simulink model "example_transient_pemfc"  (R2025a)
settings: Solver=ode15s  StartTime=0.0  StopTime=300  RelTol=1e-3
InitFcn:
  | pyenv_setup(); create_buses(5);
model workspace (MAT data in the model file):
  anFlowStruct.temperature = 344.15
  anFlowStruct.pressure = 190000
  anFlowStruct.o2 = 0
  anFlowStruct.n2 = 0
  anFlowStruct.h2 = 3.62749438e-07
  anFlowStruct.h2o = 3.83749167e-08
  anFlowStruct.liquid = 0
  caFlowStruct.temperature = 344.15
  caFlowStruct.pressure = 140000
  caFlowStruct.o2 = 2.07285393e-07
  caFlowStruct.n2 = 7.79787907e-07
  caFlowStruct.h2 = 0
  caFlowStruct.h2o = 6.4862692e-08
  caFlowStruct.liquid = 0
values from neighbouring files (symbols this model uses):
  anFlowStruct = struct('temperature', 344.15, 'pressure', 190000.,          'o2', 0., 'n2', 0., 'h2', 3.62749438e-7, 'h2o', 3.83749167e-8, 'liquid', 0.)    [build_example_transient_pemfc.m]    (also in build_transient_block.m = struct('temperature', 344.15, 'pressure', 190000.,          )
  caFlowStruct = struct('temperature', 344.15, 'pressure', 140000.,          'o2', 2.07285393e-7, 'n2', 7.79787907e-7, 'h2', 0., 'h2o', 6.48626920e-8, 'liquid', 0.)    [build_example_transient_pemfc.m]    (also in build_transient_block.m = struct('temperature', 344.15, 'pressure', 140000.,          )
settings Model: Creator=paffonsonobrega  LastModifiedBy=paffonsonobrega

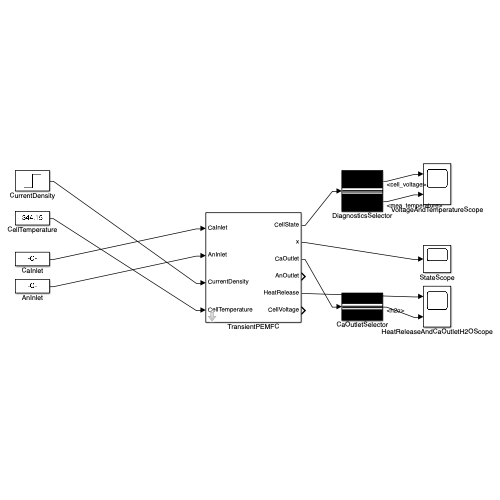
[thumbnail: Simulink's stored preview of the top-level diagram]
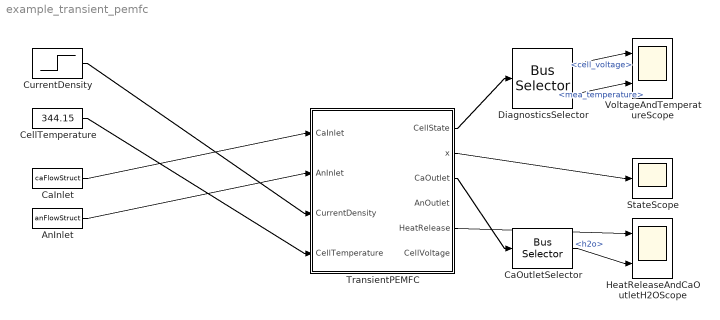
== system example_transient_pemfc ==
  AnInlet : Constant  Value=anFlowStruct  OutDataTypeStr=Bus: GasFlowStateBus
  CaInlet : Constant  Value=caFlowStruct  OutDataTypeStr=Bus: GasFlowStateBus
  CaOutletSelector : BusSelector  OutputSignals=h2o
  CellTemperature : Constant  Value=344.15
  CurrentDensity : Step  Time=100  Before=10000  After=20000  SampleTime=0
  DiagnosticsSelector : BusSelector  OutputSignals=cell_voltage,mea_temperature
  HeatReleaseAndCaOutletH2OScope : Scope  NumInputPorts=2
  StateScope : Scope
  TransientPEMFC : Subsystem  mask(TransientPEMFC){n_memb_mesh=5, cellBuilderExpr='marapendi.interop.simulink_bridge.build_default_cell', x0=[0.9783731338587631, 0.367695832038551, 0.3881598008019823, 0.40967937883127536, 0.4323084437233552, 0.4561035990835201]}
      mask prompts: n_memb_mesh "Membrane mesh nodes (n_memb_mesh)"; cellBuilderExpr "Python cell-builder function (dotted path)"; x0 "Initial ODE state x0 (1 x n_memb_mesh+1)"
      mask help:
      | Encapsulates marapendi.models.base.transient.TransientModel driven
      | directly by inlet GasFlowStates (cathode + anode) + current density
      | + cell temperature, via a Python-calling S-Function. Edit the physics
      | in the marapendi Python package; this block always calls the live model.
  VoltageAndTemperatureScope : Scope  NumInputPorts=2
  wires:
  CaInlet/1 -> TransientPEMFC/1(CaInlet)
  AnInlet/1 -> TransientPEMFC/2(AnInlet)
  CurrentDensity/1 -> TransientPEMFC/3(CurrentDensity)
  CellTemperature/1 -> TransientPEMFC/4(CellTemperature)
  TransientPEMFC/1(CellState) -> DiagnosticsSelector/1
  DiagnosticsSelector/1 -> VoltageAndTemperatureScope/1  "<cell_voltage>"
  DiagnosticsSelector/2 -> VoltageAndTemperatureScope/2  "<mea_temperature>"
  TransientPEMFC/2(x) -> StateScope/1
  TransientPEMFC/3(CaOutlet) -> CaOutletSelector/1
  TransientPEMFC/5(HeatRelease) -> HeatReleaseAndCaOutletH2OScope/1
  CaOutletSelector/1 -> HeatReleaseAndCaOutletH2OScope/2  "<h2o>"

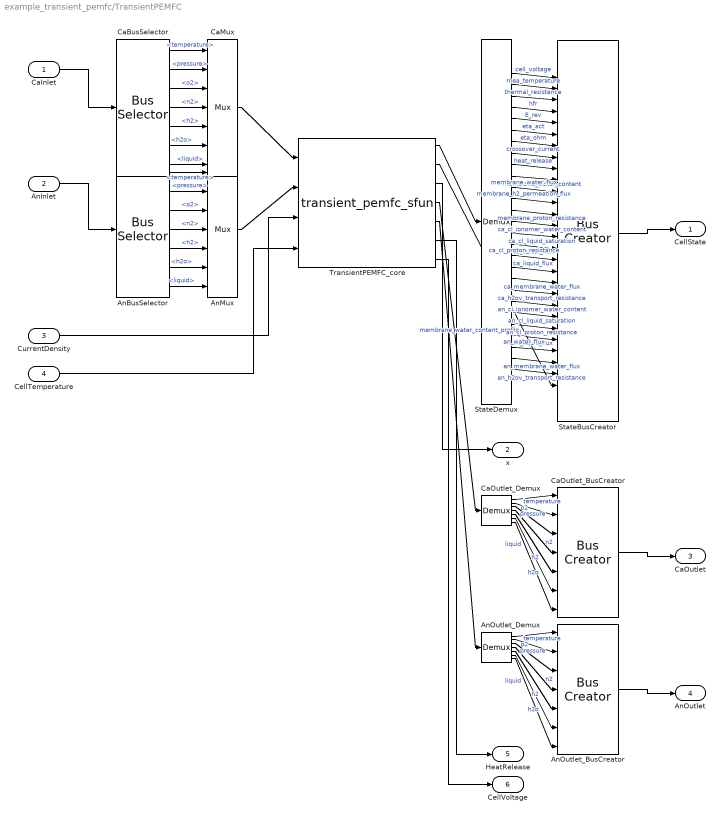
== system example_transient_pemfc/TransientPEMFC ==
  CaInlet : Inport  OutDataTypeStr=Bus: GasFlowStateBus
  AnInlet : Inport  Port=2  OutDataTypeStr=Bus: GasFlowStateBus
  CurrentDensity : Inport  Port=3
  CellTemperature : Inport  Port=4
  AnBusSelector : BusSelector  OutputSignals=temperature,pressure,o2,n2,h2,h2o,liquid
  AnMux : Mux  Inputs=7
  AnOutlet_BusCreator : BusCreator  Inputs=7  OutDataTypeStr=Bus: GasFlowStateBus  NonVirtualBus=on
  AnOutlet_Demux : Demux  Outputs=7
  CaBusSelector : BusSelector  OutputSignals=temperature,pressure,o2,n2,h2,h2o,liquid
  CaMux : Mux  Inputs=7
  CaOutlet_BusCreator : BusCreator  Inputs=7  OutDataTypeStr=Bus: GasFlowStateBus  NonVirtualBus=on
  CaOutlet_Demux : Demux  Outputs=7
  StateBusCreator : BusCreator  Inputs=28  OutDataTypeStr=Bus: CellStateBus  NonVirtualBus=on
  StateDemux : Demux  Outputs=27
  TransientPEMFC_core : M-S-Function  FunctionName=transient_pemfc_sfun  Parameters=n_memb_mesh, cellBuilderExpr, x0
  CellState : Outport
  x : Outport  Port=2
  CaOutlet : Outport  Port=3
  AnOutlet : Outport  Port=4
  HeatRelease : Outport  Port=5
  CellVoltage : Outport  Port=6
  wires:
  CaBusSelector/5 -> CaMux/5  "<h2>"
  StateBusCreator/1 -> CellState/1
  StateDemux/18 -> StateBusCreator/18  "ca_liquid_flux"
  CaBusSelector/7 -> CaMux/7  "<liquid>"
  CaBusSelector/2 -> CaMux/2  "<pressure>"
  CaMux/1 -> TransientPEMFC_core/1
  TransientPEMFC_core/7 -> CellVoltage/1
  TransientPEMFC_core/2 -> StateBusCreator/28  "membrane_water_content_profile"
  TransientPEMFC_core/4 -> CaOutlet_Demux/1
  CaBusSelector/3 -> CaMux/3  "<o2>"
  CaOutlet_BusCreator/1 -> CaOutlet/1
  AnOutlet_Demux/5 -> AnOutlet_BusCreator/5  "h2"
  StateDemux/4 -> StateBusCreator/4  "hfr"
  CaInlet/1 -> CaBusSelector/1
  AnInlet/1 -> AnBusSelector/1
  CurrentDensity/1 -> TransientPEMFC_core/3
  CaBusSelector/6 -> CaMux/6  "<h2o>"
  StateDemux/15 -> StateBusCreator/15  "ca_cl_liquid_saturation"
  AnOutlet_Demux/6 -> AnOutlet_BusCreator/6  "h2o"
  AnBusSelector/7 -> AnMux/7  "<liquid>"
  StateDemux/22 -> StateBusCreator/22  "an_cl_liquid_saturation"
  AnBusSelector/5 -> AnMux/5  "<h2>"
  AnMux/1 -> TransientPEMFC_core/2
  AnOutlet_Demux/4 -> AnOutlet_BusCreator/4  "n2"
  TransientPEMFC_core/1 -> StateDemux/1
  AnBusSelector/4 -> AnMux/4  "<n2>"
  CaBusSelector/1 -> CaMux/1  "<temperature>"
  StateDemux/17 -> StateBusCreator/17  "ca_water_flux"
  StateDemux/19 -> StateBusCreator/19  "ca_membrane_water_flux"
  CellTemperature/1 -> TransientPEMFC_core/4
  StateDemux/23 -> StateBusCreator/23  "an_cl_proton_resistance"
  AnBusSelector/3 -> AnMux/3  "<o2>"
  CaBusSelector/4 -> CaMux/4  "<n2>"
  StateDemux/9 -> StateBusCreator/9  "heat_release"
  StateDemux/12 -> StateBusCreator/12  "membrane_h2_permeation_flux"
  CaOutlet_Demux/5 -> CaOutlet_BusCreator/5  "h2"
  StateDemux/1 -> StateBusCreator/1  "cell_voltage"
  StateDemux/14 -> StateBusCreator/14  "ca_cl_ionomer_water_content"
  StateDemux/10 -> StateBusCreator/10  "membrane_water_content"
  TransientPEMFC_core/5 -> AnOutlet_Demux/1
  AnBusSelector/6 -> AnMux/6  "<h2o>"
  CaOutlet_Demux/7 -> CaOutlet_BusCreator/7  "liquid"
  StateDemux/8 -> StateBusCreator/8  "crossover_current"
  CaOutlet_Demux/4 -> CaOutlet_BusCreator/4  "n2"
  AnOutlet_Demux/7 -> AnOutlet_BusCreator/7  "liquid"
  TransientPEMFC_core/3 -> x/1
  AnOutlet_BusCreator/1 -> AnOutlet/1
  StateDemux/13 -> StateBusCreator/13  "membrane_proton_resistance"
  StateDemux/11 -> StateBusCreator/11  "membrane_water_flux"
  StateDemux/7 -> StateBusCreator/7  "eta_ohm"
  AnBusSelector/2 -> AnMux/2  "<pressure>"
  AnOutlet_Demux/3 -> AnOutlet_BusCreator/3  "o2"
  StateDemux/5 -> StateBusCreator/5  "E_rev"
  StateDemux/2 -> StateBusCreator/2  "mea_temperature"
  StateDemux/26 -> StateBusCreator/26  "an_membrane_water_flux"
  StateDemux/27 -> StateBusCreator/27  "an_h2ov_transport_resistance"
  CaOutlet_Demux/6 -> CaOutlet_BusCreator/6  "h2o"
  StateDemux/3 -> StateBusCreator/3  "thermal_resistance"
  StateDemux/25 -> StateBusCreator/25  "an_liquid_flux"
  StateDemux/24 -> StateBusCreator/24  "an_water_flux"
  StateDemux/20 -> StateBusCreator/20  "ca_h2ov_transport_resistance"
  StateDemux/21 -> StateBusCreator/21  "an_cl_ionomer_water_content"
  CaOutlet_Demux/3 -> CaOutlet_BusCreator/3  "o2"
  AnBusSelector/1 -> AnMux/1  "<temperature>"
  StateDemux/16 -> StateBusCreator/16  "ca_cl_proton_resistance"
  AnOutlet_Demux/1 -> AnOutlet_BusCreator/1  "temperature"
  StateDemux/6 -> StateBusCreator/6  "eta_act"
  CaOutlet_Demux/1 -> CaOutlet_BusCreator/1  "temperature"
  CaOutlet_Demux/2 -> CaOutlet_BusCreator/2  "pressure"
  AnOutlet_Demux/2 -> AnOutlet_BusCreator/2  "pressure"
  TransientPEMFC_core/6 -> HeatRelease/1
